simulink subsystem "LowContr"  (R2023a)
settings: Solver=VariableStepAuto  StartTime=0.0  StopTime=10.0  RelTol=1e-3
settings Model: Creator=lehas  LastModifiedBy=lehas

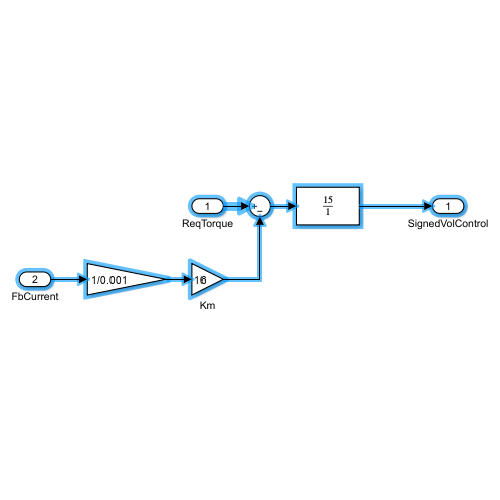
[thumbnail: Simulink's stored preview of the top-level diagram]
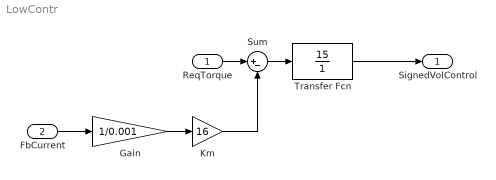
== system LowContr ==
  ReqTorque : Inport
  FbCurrent : Inport  Port=2
  Gain : Gain  Gain=1/0.001
  Km : Gain  Gain=16
  Sum : Sum  Inputs=|+-
  Transfer Fcn : TransferFcn  Numerator=[15]  Denominator=[1]
  SignedVolControl : Outport
  wires:
  Km/1 -> Sum/2
  Sum/1 -> Transfer Fcn/1
  Gain/1 -> Km/1
  Transfer Fcn/1 -> SignedVolControl/1
  FbCurrent/1 -> Gain/1
  ReqTorque/1 -> Sum/1
